simulink model "Pitch_shift_HDL"  (R2018b)
settings: Solver=FixedStepDiscrete  StartTime=0.0  StopTime=5  RelTol=1e-3
InitFcn:
  | load speech_signal
  | Fs = 48000;
  | Ts = 1/Fs;
  | 
  | FFT_size = 128;
  | FFT_size_half = FFT_size/2;
  | FFT_frame_shift = FFT_size/4;  % should be a power of two (to easily replace mode operator that is not HDL compatible)
  | FFT_frame_shift_Nbits = log2(FFT_frame_shift);
  | 
  | DPRAM1_size = FFT_size*2;  % number of words
  | DPRAM1_address_size = log2(DPRAM1_size);
  | 
  | 
  | 
  | SysRate_Upsample_Factor = 32;
  | 
  | 
  | Wbits = 32;    %fixdt(1,Wbits,Fbits)
  | Fbits = 28;
libraries: hdlsllib x16, simulink x5, dspxfrm3 x2, dspsigops x2
settings Model: Creator=Ross_admin  LastModifiedBy=Ross
settings OptimizationCC: BlockReduction=off  ConditionallyExecuteInputs=off  DefaultParameterBehavior=Inlined
settings DebuggingCC: AlgebraicLoopMsg=error  SingleTaskRateTransMsg=error
settings HardwareCC: ProdBitPerPointer=32  ProdBitPerSizeT=32  ProdBitPerPtrDiffT=32  ProdLargestAtomicFloat=None  ProdIntDivRoundTo=Undefined  ProdEndianess=Unspecified  ProdWordSize=32  ProdHWDeviceType=ASIC/FPGA->ASIC/FPGA  TargetBitPerPointer=64  TargetBitPerSizeT=64  TargetBitPerPtrDiffT=64  TargetLongLongMode=on  TargetIntDivRoundTo=Zero  TargetEndianess=LittleEndian  TargetWordSize=64  TargetHWDeviceType=Custom Processor->MATLAB Host Computer  ProdEqTarget=off
settings SFSimCC: SimUseLocalCustomCode=off
settings RTWCC: RTWUseLocalCustomCode=off
settings CodeAppCC: StateflowObjectComments=on

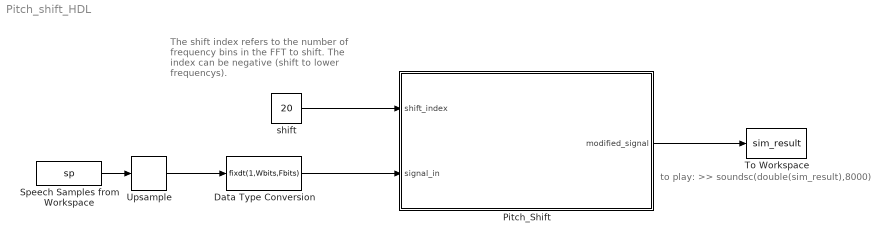
== system Pitch_shift_HDL ==
  note: The shift index refers to the number of
      | frequency bins in the FFT to shift.
      | The index can be negative
      | (shift to lower frequencys).
  note: to play: >> soundsc(double(sim_result),8000)
  Data Type Conversion : DataTypeConversion  OutDataTypeStr=fixdt(1,Wbits,Fbits)
  Pitch_Shift : Subsystem  TreatAsAtomicUnit=on
  Speech Samples from Workspace : FromWorkspace  VariableName=sp  SampleTime=Ts*6
  To Workspace : ToWorkspace  VariableName=sim_result  SampleTime=-1
  Upsample : dspsigops/Upsample  N=6  phase=0  RateOptions=Allow multirate processing  ic=0  mode=Unused parameter value
  shift : Constant  Value=20  OutDataTypeStr=fixdt(1,16,0)  SampleTime=Ts
  wires:
  Speech Samples from Workspace/1 -> Upsample/1
  Pitch_Shift/1(modified_signal) -> To Workspace/1
  Data Type Conversion/1 -> Pitch_Shift/2(signal_in)
  Upsample/1 -> Data Type Conversion/1
  shift/1 -> Pitch_Shift/1(shift_index)

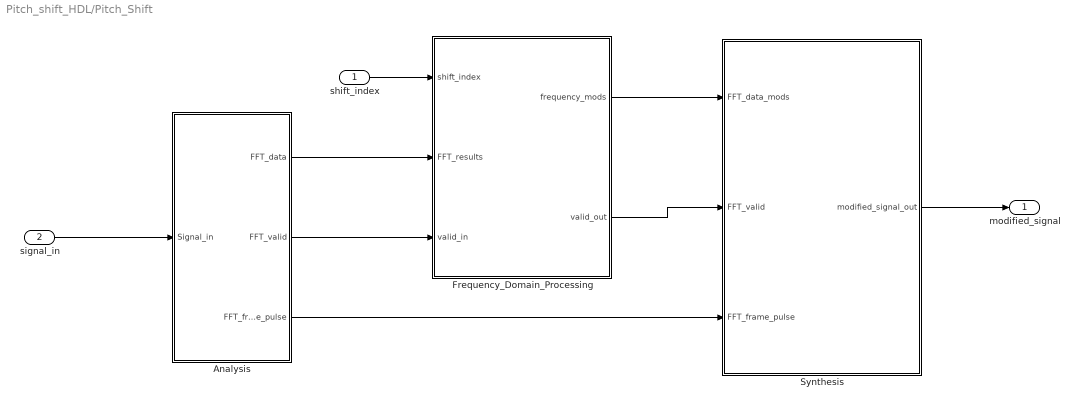
== system Pitch_shift_HDL/Pitch_Shift ==
  shift_index : Inport
  signal_in : Inport  Port=2
  Analysis : Subsystem
  Frequency_Domain_Processing : Subsystem
  Synthesis : Subsystem
  modified_signal : Outport
  wires:
  shift_index/1 -> Frequency_Domain_Processing/1(shift_index)
  signal_in/1 -> Analysis/1(Signal_in)
  Analysis/1(FFT_data) -> Frequency_Domain_Processing/2(FFT_results)
  Analysis/2(FFT_valid) -> Frequency_Domain_Processing/3(valid_in)
  Frequency_Domain_Processing/1(frequency_mods) -> Synthesis/1(FFT_data_mods)
  Frequency_Domain_Processing/2(valid_out) -> Synthesis/2(FFT_valid)
  Analysis/3(FFT_frame_pulse) -> Synthesis/3(FFT_frame_pulse)
  Synthesis/1(modified_signal_out) -> modified_signal/1

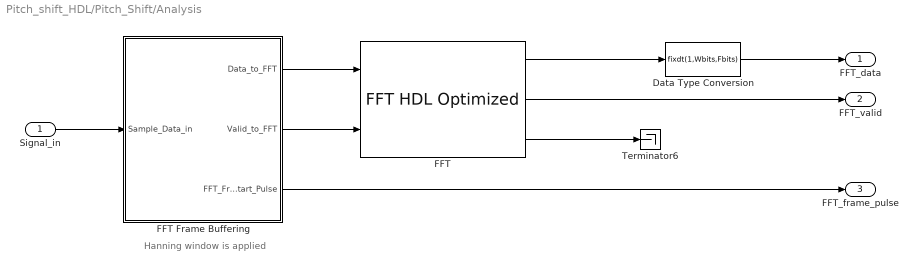
== system Pitch_shift_HDL/Pitch_Shift/Analysis ==
  note: Hanning window is applied
  Signal_in : Inport
  Data Type Conversion : DataTypeConversion  OutDataTypeStr=fixdt(1,Wbits,Fbits)
  FFT : dspxfrm3/FFT HDL Optimized  FFTLength=FFT_size  Architecture=Burst Radix 2  ComplexMultiplication=Use 4 multipliers and 2 adders  BitReversedOutput=off  BitReversedInput=off  Normalize=off  SimulateUsing=Code generation  RoundingMethod=Floor  ResetInputPort=off  StartOutputPort=off  EndOutputPort=off
      settings: SourceProductName=DSP System Toolbox  SourceProductBaseCode=DS
  FFT Frame Buffering : Subsystem
  Terminator6 : Terminator
  FFT_data : Outport
  FFT_valid : Outport  Port=2
  FFT_frame_pulse : Outport  Port=3
  wires:
  FFT/3 -> Terminator6/1
  FFT Frame Buffering/3(FFT_Frame_Start_Pulse) -> FFT_frame_pulse/1
  Signal_in/1 -> FFT Frame Buffering/1(Sample_Data_in)
  FFT Frame Buffering/2(Valid_to_FFT) -> FFT/2
  FFT Frame Buffering/1(Data_to_FFT) -> FFT/1
  Data Type Conversion/1 -> FFT_data/1
  FFT/2 -> FFT_valid/1
  FFT/1 -> Data Type Conversion/1

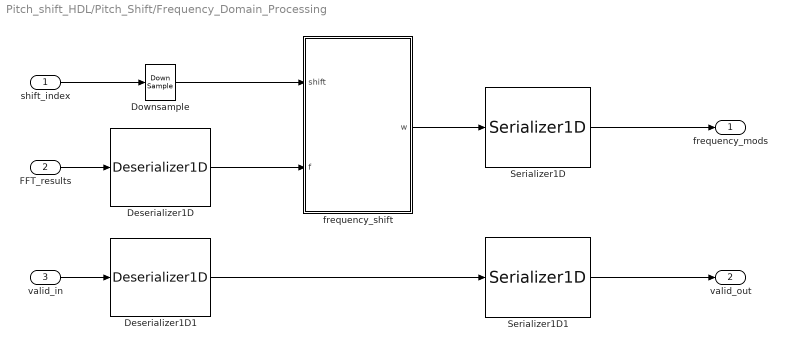
== system Pitch_shift_HDL/Pitch_Shift/Frequency_Domain_Processing ==
  shift_index : Inport
  FFT_results : Inport  Port=2
  valid_in : Inport  Port=3
  Deserializer1D : hdlsllib/HDL Operations/Deserializer1D  Ratio=FFT_size  IdleCycles=0  InitialCondition=0  startIn=off  validIn=off  validOut=off  inputDataDimensions=-1  inputSampleTime=-1  inputSignalType=auto
      settings: SourceProductName=HDL Coder  SourceProductBaseCode=HD
  Deserializer1D1 : hdlsllib/HDL Operations/Deserializer1D  Ratio=FFT_size  IdleCycles=0  InitialCondition=0  startIn=off  validIn=off  validOut=off  inputDataDimensions=-1  inputSampleTime=-1  inputSignalType=auto
      settings: SourceProductName=HDL Coder  SourceProductBaseCode=HD
  Downsample : DownSample  N=FFT_size/SysRate_Upsample_Factor  RateOptions=Allow multirate processing
  Serializer1D : hdlsllib/HDL Operations/Serializer1D  Ratio=FFT_size  IdleCycles=0  validIn=off  startOut=off  validOut=off  inputDataDimensions=-1  inputSampleTime=-1  inputSignalType=auto
      settings: SourceProductName=HDL Coder  SourceProductBaseCode=HD
  Serializer1D1 : hdlsllib/HDL Operations/Serializer1D  Ratio=FFT_size  IdleCycles=0  validIn=off  startOut=off  validOut=off  inputDataDimensions=-1  inputSampleTime=-1  inputSignalType=auto
      settings: SourceProductName=HDL Coder  SourceProductBaseCode=HD
  frequency_shift : MATLAB Function  TreatAsAtomicUnit=on
  frequency_mods : Outport
  valid_out : Outport  Port=2
  wires:
  Deserializer1D1/1 -> Serializer1D1/1
  Deserializer1D/1 -> frequency_shift/2(f)
  FFT_results/1 -> Deserializer1D/1
  frequency_shift/1(w) -> Serializer1D/1
  Serializer1D/1 -> frequency_mods/1
  valid_in/1 -> Deserializer1D1/1
  shift_index/1 -> Downsample/1
  Serializer1D1/1 -> valid_out/1
  Downsample/1 -> frequency_shift/1(shift)

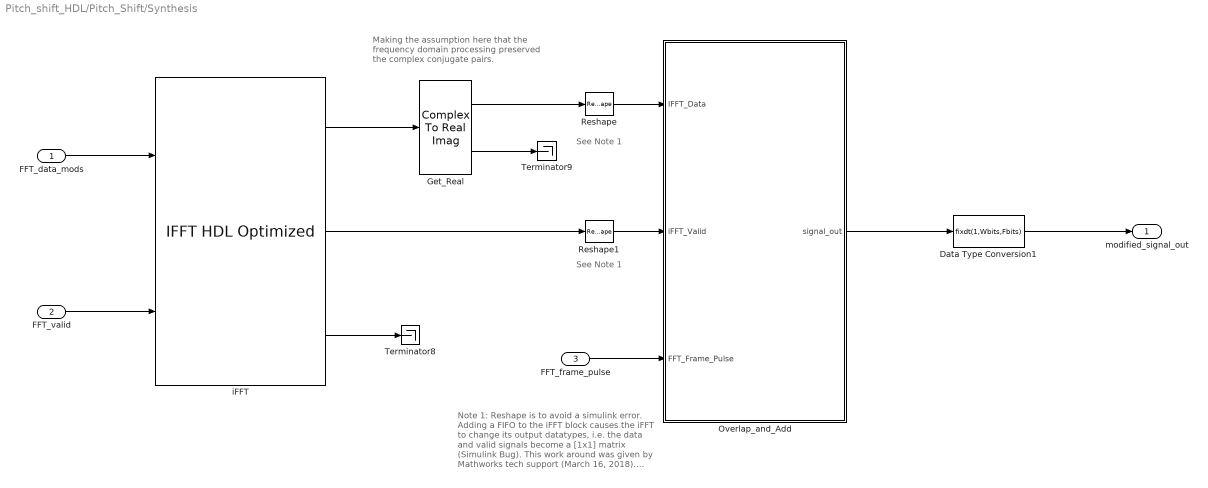
== system Pitch_shift_HDL/Pitch_Shift/Synthesis ==
  note: Making the assumption here
      | that the frequency domain processing
      | preserved the complex conjugate pairs.
  note: See Note 1
  note: Note 1:
      | Reshape is to avoid a simulink error.
      | Adding a FIFO to the iFFT block causes the
      | iFFT to change its output datatypes,
      | i.e. the data and valid signals
      | become a [1x1] matrix (Simulink Bug).
      | This work around was given by Mathworks
      | tech support (March 16, 2018).
      | Matlab 2017b
  note: See Note 1
  FFT_data_mods : Inport
  FFT_valid : Inport  Port=2
  FFT_frame_pulse : Inport  Port=3
  Data Type Conversion1 : DataTypeConversion  OutDataTypeStr=fixdt(1,Wbits,Fbits)
  Get_Real : ComplexToRealImag
  Overlap_and_Add : Subsystem
  Reshape : Reshape
  Reshape1 : Reshape
  Terminator8 : Terminator
  Terminator9 : Terminator
  iFFT : dspxfrm3/IFFT HDL Optimized  FFTLength=FFT_size  Architecture=Burst Radix 2  ComplexMultiplication=Use 4 multipliers and 2 adders  BitReversedOutput=off  BitReversedInput=off  Normalize=on  SimulateUsing=Code generation  RoundingMethod=Floor  ResetInputPort=off  StartOutputPort=off  EndOutputPort=off
      settings: SourceProductName=DSP System Toolbox  SourceProductBaseCode=DS
  modified_signal_out : Outport
  wires:
  iFFT/3 -> Terminator8/1
  Reshape1/1 -> Overlap_and_Add/2(iFFT_Valid)
  Reshape/1 -> Overlap_and_Add/1(IFFT_Data)
  iFFT/2 -> Reshape1/1
  Overlap_and_Add/1(signal_out) -> Data Type Conversion1/1
  FFT_data_mods/1 -> iFFT/1
  Data Type Conversion1/1 -> modified_signal_out/1
  iFFT/1 -> Get_Real/1
  Get_Real/1 -> Reshape/1
  Get_Real/2 -> Terminator9/1
  FFT_valid/1 -> iFFT/2
  FFT_frame_pulse/1 -> Overlap_and_Add/3(FFT_Frame_Pulse)

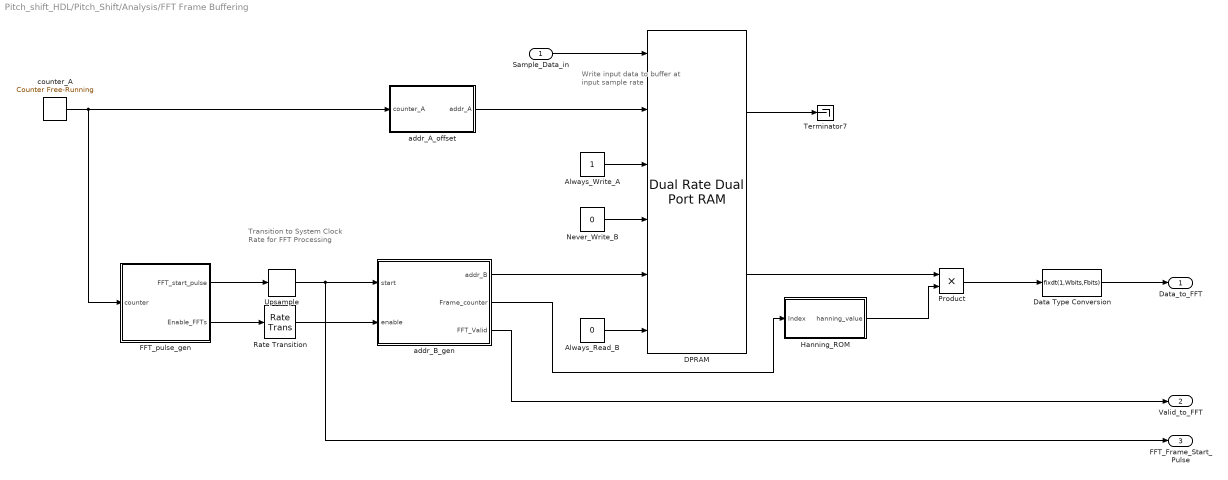
== system Pitch_shift_HDL/Pitch_Shift/Analysis/FFT Frame Buffering ==
  note: Transition to
      | System Clock Rate
      | for FFT Processing
  note: Write input data
      | to buffer at input
      | sample rate
  Sample_Data_in : Inport
  Always_Read_B : Constant  Value=0  OutDataTypeStr=boolean  SampleTime=Ts/SysRate_Upsample_Factor
  Always_Write_A : Constant  OutDataTypeStr=boolean  SampleTime=Ts
  DPRAM : hdlsllib/HDL RAMs/Dual Rate Dual Port RAM  ram_size=DPRAM1_address_size
      settings: SourceProductName=HDL Coder  SourceProductBaseCode=HD
  Data Type Conversion : DataTypeConversion  OutDataTypeStr=fixdt(1,Wbits,Fbits)
  FFT_pulse_gen : Subsystem
  Hanning_ROM : Subsystem
  Never_Write_B : Constant  Value=0  OutDataTypeStr=fixdt(1,Wbits,Fbits)  SampleTime=Ts/SysRate_Upsample_Factor
  Product : Product
  Rate Transition : RateTransition  OutPortSampleTimeOpt=Multiple of input port sample time  OutPortSampleTimeMultiple=1/SysRate_Upsample_Factor
  Terminator7 : Terminator
  Upsample : dspsigops/Upsample  N=SysRate_Upsample_Factor  phase=0  RateOptions=Allow multirate processing  ic=0  mode=Unused parameter value
  addr_A_offset : Subsystem
  addr_B_gen : Subsystem
  counter_A : simulink/Sources/Counter Free-Running  NumBits=DPRAM1_address_size  tsamp=Ts
  Data_to_FFT : Outport
  Valid_to_FFT : Outport  Port=2
  FFT_Frame_Start_Pulse : Outport  Port=3
  wires:
  Always_Write_A/1 -> DPRAM/3
  Never_Write_B/1 -> DPRAM/4
  Always_Read_B/1 -> DPRAM/6
  DPRAM/1 -> Terminator7/1
  addr_B_gen/3(FFT_Valid) -> Valid_to_FFT/1
  addr_B_gen/1(addr_B) -> DPRAM/5
  counter_A/1 -> addr_A_offset/1(counter_A), FFT_pulse_gen/1(counter)
  Sample_Data_in/1 -> DPRAM/1
  addr_A_offset/1(addr_A) -> DPRAM/2
  addr_B_gen/2(Frame_counter) -> Hanning_ROM/1(Index)
  Product/1 -> Data Type Conversion/1
  DPRAM/2 -> Product/1
  Hanning_ROM/1(hanning_value) -> Product/2
  Data Type Conversion/1 -> Data_to_FFT/1
  Rate Transition/1 -> addr_B_gen/2(enable)
  FFT_pulse_gen/1(FFT_start_pulse) -> Upsample/1
  FFT_pulse_gen/2(Enable_FFTs) -> Rate Transition/1
  Upsample/1 -> FFT_Frame_Start_Pulse/1, addr_B_gen/1(start)

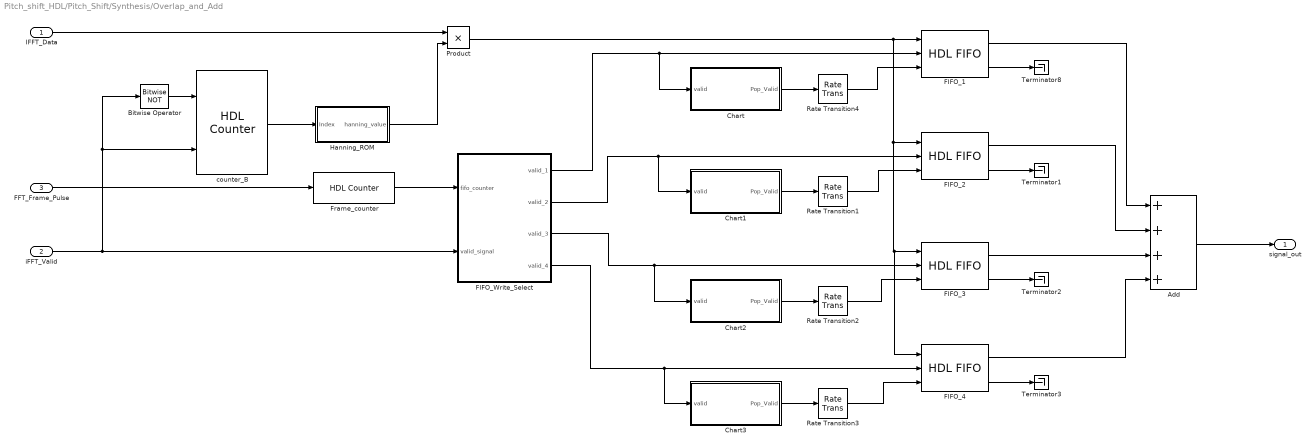
== system Pitch_shift_HDL/Pitch_Shift/Synthesis/Overlap_and_Add ==
  IFFT_Data : Inport
  iFFT_Valid : Inport  Port=2
  FFT_Frame_Pulse : Inport  Port=3
  Add : Sum  Inputs=4
  Bitwise Operator : simulink/Logic and Bit Operations/Bitwise Operator  logicop=NOT  UseBitMask=off  BitMask=bin2dec('11011001')  BitMaskRealWorld=Stored Integer
  Chart : Stateflow chart  TreatAsAtomicUnit=on
  Chart1 : Stateflow chart  TreatAsAtomicUnit=on
  Chart2 : Stateflow chart  TreatAsAtomicUnit=on
  Chart3 : Stateflow chart  TreatAsAtomicUnit=on
  FIFO_{1..4} (4 alike) : hdlsllib/HDL RAMs/HDL FIFO  fifo_size=FFT_size  ratio=SysRate_Upsample_Factor  push_msg=Warning  pop_msg=Warning  show_empty=off  show_full=on  show_num=off
      settings: SourceProductName=HDL Coder  SourceProductBaseCode=HD
  FIFO_Write_Select : MATLAB Function  TreatAsAtomicUnit=on
  Frame_counter : hdlsllib/Sources/HDL Counter  CountType=Free running  CountInit=2  CountStep=1  CountMax=1024  CountFromType=Initial value  CountFrom=2  CountResetPort=off  CountLoadPort=off  CountEnbPort=on  CountDirPort=off  CountDataType=Unsigned  CountWordLen=2  CountFracLen=0  CountSampTime=1
      settings: SourceProductBaseCode=HD
  Hanning_ROM : Subsystem
  Product : Product
  Rate Transition{1..4} (4 alike) : RateTransition  OutPortSampleTimeOpt=Multiple of input port sample time  OutPortSampleTimeMultiple=SysRate_Upsample_Factor
  Terminator{1..3,8} (4 alike) : Terminator
  counter_B : hdlsllib/Sources/HDL Counter  CountType=Count limited  CountInit=0  CountStep=1  CountMax=FFT_size  CountFromType=Initial value  CountFrom=0  CountResetPort=on  CountLoadPort=off  CountEnbPort=on  CountDirPort=off  CountDataType=Unsigned  CountWordLen=DPRAM1_address_size  CountFracLen=0  CountSampTime=1
      settings: SourceProductBaseCode=HD
  signal_out : Outport
  wires:
  FIFO_1/1 -> Add/1
  FIFO_3/1 -> Add/3
  FFT_Frame_Pulse/1 -> Frame_counter/1
  FIFO_2/1 -> Add/2
  FIFO_Write_Select/3(valid_3) -> Chart2/1(valid), FIFO_3/2
  FIFO_Write_Select/4(valid_4) -> Chart3/1(valid), FIFO_4/2
  FIFO_4/1 -> Add/4
  FIFO_Write_Select/1(valid_1) -> FIFO_1/2, Chart/1(valid)
  FIFO_Write_Select/2(valid_2) -> FIFO_2/2, Chart1/1(valid)
  Add/1 -> signal_out/1
  Frame_counter/1 -> FIFO_Write_Select/1(fifo_counter)
  FIFO_4/2 -> Terminator3/1
  FIFO_2/2 -> Terminator1/1
  FIFO_3/2 -> Terminator2/1
  Bitwise Operator/1 -> counter_B/1
  iFFT_Valid/1 -> counter_B/2, Bitwise Operator/1, FIFO_Write_Select/2(valid_signal)
  IFFT_Data/1 -> Product/1
  Product/1 -> FIFO_4/1, FIFO_3/1, FIFO_2/1, FIFO_1/1
  Hanning_ROM/1(hanning_value) -> Product/2
  counter_B/1 -> Hanning_ROM/1(Index)
  Chart/1(Pop_Valid) -> Rate Transition4/1
  Rate Transition4/1 -> FIFO_1/3
  FIFO_1/2 -> Terminator8/1
  Chart1/1(Pop_Valid) -> Rate Transition1/1
  Rate Transition1/1 -> FIFO_2/3
  Chart2/1(Pop_Valid) -> Rate Transition2/1
  Rate Transition2/1 -> FIFO_3/3
  Chart3/1(Pop_Valid) -> Rate Transition3/1
  Rate Transition3/1 -> FIFO_4/3

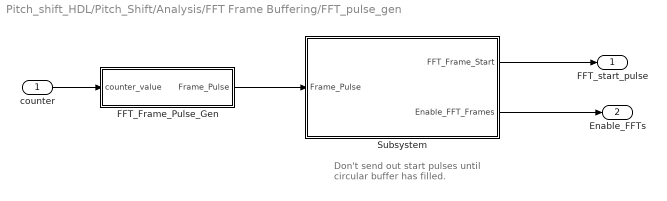
== system Pitch_shift_HDL/Pitch_Shift/Analysis/FFT Frame Buffering/FFT_pulse_gen ==
  note: Don't send out start pulses until
      | circular buffer has filled.
  counter : Inport
  FFT_Frame_Pulse_Gen : Subsystem
  Subsystem : Subsystem
  FFT_start_pulse : Outport
  Enable_FFTs : Outport  Port=2
  wires:
  counter/1 -> FFT_Frame_Pulse_Gen/1("counter_value ")
  Subsystem/1(FFT_Frame_Start) -> FFT_start_pulse/1
  Subsystem/2(Enable_FFT_Frames) -> Enable_FFTs/1
  FFT_Frame_Pulse_Gen/1(Frame_Pulse) -> Subsystem/1(Frame_Pulse)

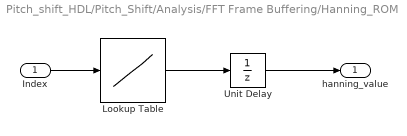
== system Pitch_shift_HDL/Pitch_Shift/Analysis/FFT Frame Buffering/Hanning_ROM ==
  Index : Inport
  Lookup Table : Lookup_n-D  NumberOfTableDimensions=1  BreakpointsForDimension1=[0:FFT_size]  IndexSearchMethod=Evenly spaced points  Table=hanning(FFT_size+1)  InterpMethod=Flat  ExtrapMethod=Clip  DiagnosticForOutOfRangeInput=Error  UseLastTableValue=on  OutDataTypeStr=fixdt(1,24,22)  RndMeth=Simplest  InputSameDT=on
  Unit Delay : UnitDelay  SampleTime=-1
  hanning_value : Outport
  wires:
  Unit Delay/1 -> hanning_value/1
  Index/1 -> Lookup Table/1
  Lookup Table/1 -> Unit Delay/1

== system Pitch_shift_HDL/Pitch_Shift/Analysis/FFT Frame Buffering/addr_A_offset ==
  note: Add 1 to counter since the read pointer (addr_B)
      | can catch the write pointer (addr_A) if
      | SysRate_Upsample_Factor is large enough
  counter_A : Inport
  Add : Sum  OutDataTypeStr=fixdt(0,DPRAM1_address_size,0)
  write_offset : Constant  OutDataTypeStr=fixdt(0,DPRAM1_address_size,0)  SampleTime=Ts
  addr_A : Outport
  wires:
  write_offset/1 -> Add/2
  Add/1 -> addr_A/1
  counter_A/1 -> Add/1

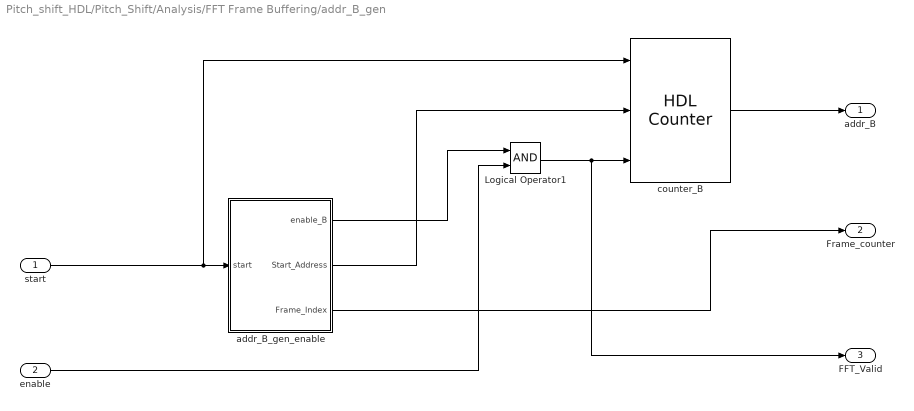
== system Pitch_shift_HDL/Pitch_Shift/Analysis/FFT Frame Buffering/addr_B_gen ==
  start : Inport
  enable : Inport  Port=2
  Logical Operator1 : Logic  AllPortsSameDT=off  OutDataTypeStr=boolean
  addr_B_gen_enable : Subsystem
  counter_B : hdlsllib/Sources/HDL Counter  CountType=Free running  CountInit=DPRAM1_size-10  CountStep=1  CountMax=1024  CountFromType=Initial value  CountFrom=DPRAM1_size-10  CountResetPort=off  CountLoadPort=on  CountEnbPort=on  CountDirPort=off  CountDataType=Unsigned  CountWordLen=DPRAM1_address_size  CountFracLen=0  CountSampTime=1
      settings: SourceProductBaseCode=HD
  addr_B : Outport
  Frame_counter : Outport  Port=2
  FFT_Valid : Outport  Port=3
  wires:
  counter_B/1 -> addr_B/1
  start/1 -> counter_B/1, addr_B_gen_enable/1(start)
  addr_B_gen_enable/1(enable_B) -> Logical Operator1/1
  addr_B_gen_enable/2(Start_Address) -> counter_B/2
  enable/1 -> Logical Operator1/2
  addr_B_gen_enable/3(Frame_Index) -> Frame_counter/1
  Logical Operator1/1 -> FFT_Valid/1, counter_B/3

== system Pitch_shift_HDL/Pitch_Shift/Synthesis/Overlap_and_Add/Hanning_ROM ==
  Index : Inport
  Lookup Table : Lookup_n-D  NumberOfTableDimensions=1  BreakpointsForDimension1=[0:FFT_size]  IndexSearchMethod=Evenly spaced points  Table=hanning(FFT_size+1)  InterpMethod=Flat  ExtrapMethod=Clip  DiagnosticForOutOfRangeInput=Error  UseLastTableValue=on  OutDataTypeStr=fixdt(1,24,22)  RndMeth=Simplest  InputSameDT=on
  Unit Delay : UnitDelay  SampleTime=-1
  hanning_value : Outport
  wires:
  Unit Delay/1 -> hanning_value/1
  Index/1 -> Lookup Table/1
  Lookup Table/1 -> Unit Delay/1

== system Pitch_shift_HDL/Pitch_Shift/Analysis/FFT Frame Buffering/FFT_pulse_gen/FFT_Frame_Pulse_Gen ==
  "counter_value " : Inport
  Bit Slice : hdlsllib/Logic and Bit Operations/Bit Slice  lidx=log2(FFT_frame_shift)-1  ridx=0
  Compare To Zero : simulink/Logic and Bit Operations/Compare To Zero  relop===  OutDataTypeStr=boolean
  Frame_Pulse : Outport
  wires:
  "counter_value "/1 -> Bit Slice/1
  Compare To Zero/1 -> Frame_Pulse/1
  Bit Slice/1 -> Compare To Zero/1

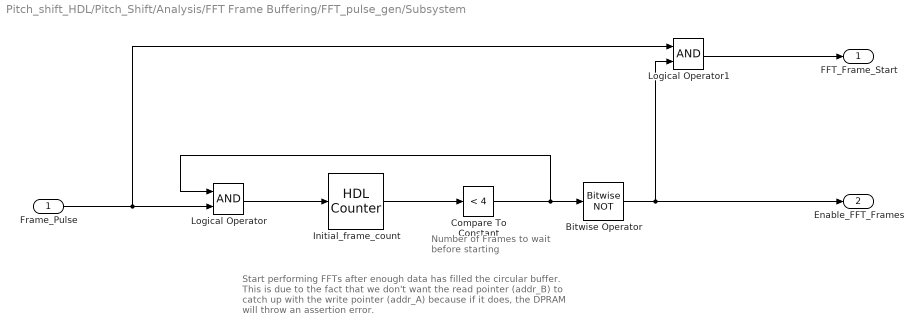
== system Pitch_shift_HDL/Pitch_Shift/Analysis/FFT Frame Buffering/FFT_pulse_gen/Subsystem ==
  note: Number of Frames
      | to wait before starting
  note: Start performing FFTs after enough data has filled the circular buffer.
      | This is due to the fact that we don't want the read pointer (addr_B)
      | to catch up with the  write pointer (addr_A) because if it does,
      | the DPRAM will throw an assertion error.
  Frame_Pulse : Inport
  Bitwise Operator : simulink/Logic and Bit Operations/Bitwise Operator  logicop=NOT  UseBitMask=off  BitMask=bin2dec('11011001')  BitMaskRealWorld=Stored Integer
  Compare To Constant : simulink/Logic and Bit Operations/Compare To Constant  relop=<  const=4  OutDataTypeStr=boolean
  Initial_frame_count : hdlsllib/Sources/HDL Counter  CountType=Count limited  CountInit=0  CountStep=1  CountMax=4  CountFromType=Specify  CountFrom=0  CountResetPort=off  CountLoadPort=off  CountEnbPort=on  CountDirPort=off  CountDataType=Unsigned  CountWordLen=5  CountFracLen=0  CountSampTime=1
      settings: SourceProductBaseCode=HD
  Logical Operator : Logic  AllPortsSameDT=off  OutDataTypeStr=boolean
  Logical Operator1 : Logic  AllPortsSameDT=off  OutDataTypeStr=boolean
  FFT_Frame_Start : Outport
  Enable_FFT_Frames : Outport  Port=2
  wires:
  Logical Operator1/1 -> FFT_Frame_Start/1
  Frame_Pulse/1 -> Logical Operator/2, Logical Operator1/1
  Initial_frame_count/1 -> Compare To Constant/1
  Logical Operator/1 -> Initial_frame_count/1
  Compare To Constant/1 -> Bitwise Operator/1, Logical Operator/1
  Bitwise Operator/1 -> Enable_FFT_Frames/1, Logical Operator1/2

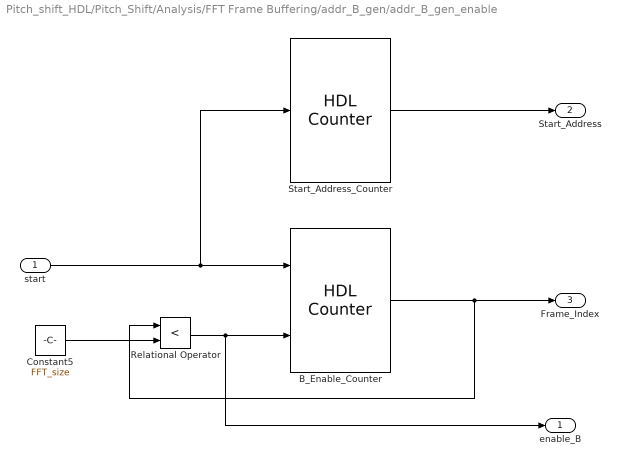
== system Pitch_shift_HDL/Pitch_Shift/Analysis/FFT Frame Buffering/addr_B_gen/addr_B_gen_enable ==
  start : Inport
  B_Enable_Counter : hdlsllib/Sources/HDL Counter  CountType=Count limited  CountInit=0  CountStep=1  CountMax=FFT_size  CountFromType=Specify  CountFrom=0  CountResetPort=on  CountLoadPort=off  CountEnbPort=on  CountDirPort=off  CountDataType=Unsigned  CountWordLen=DPRAM1_address_size  CountFracLen=0  CountSampTime=1
      settings: SourceProductBaseCode=HD
  Constant5 : Constant  Value=FFT_size  OutDataTypeStr=fixdt(0,11,0)  SampleTime=Ts/SysRate_Upsample_Factor
  Relational Operator : RelationalOperator  Operator=<  OutDataTypeStr=boolean  ZeroCross=off  RndMeth=Nearest
  Start_Address_Counter : hdlsllib/Sources/HDL Counter  CountType=Free running  CountInit=0  CountStep=FFT_frame_shift  CountMax=DPRAM1_size  CountFromType=Initial value  CountFrom=0  CountResetPort=off  CountLoadPort=off  CountEnbPort=on  CountDirPort=off  CountDataType=Unsigned  CountWordLen=DPRAM1_address_size  CountFracLen=0  CountSampTime=1
      settings: SourceProductBaseCode=HD
  enable_B : Outport
  Start_Address : Outport  Port=2
  Frame_Index : Outport  Port=3
  wires:
  Relational Operator/1 -> enable_B/1, B_Enable_Counter/2
  Constant5/1 -> Relational Operator/2
  B_Enable_Counter/1 -> Frame_Index/1, Relational Operator/1
  start/1 -> Start_Address_Counter/1, B_Enable_Counter/1
  Start_Address_Counter/1 -> Start_Address/1

== stateflow chart Pitch_shift_HDL/Pitch_Shift/Synthesis/Overlap_and_Add/Chart1 ==
  settings: executeAtInitialization=1
  state valid_high
    entry: Pop_Valid=fi(0,0,1,0);
  state Pop_assert
    entry: Pop_Valid=fi(1,0,1,0);
  state valid_low
    entry: Pop_Valid=fi(0,0,1,0);
  state Start_up
    entry: Pop_Valid=fi(0,0,1,0);
  (default) -> Start_up
  Start_up -> valid_low : [valid == 0]
  valid_high -> Pop_assert [order 1] : [valid == 0]
  valid_low -> valid_high [order 1] : [valid == 1]
  valid_low -> valid_low [order 2] : [valid == 0]
  valid_high -> valid_high [order 2] : [valid == 1]
  data: valid input; Pop_Valid output

== matlab function Pitch_shift_HDL/Pitch_Shift/Synthesis/Overlap_and_Add/FIFO_Write_Select ==
  data: fifo_counter input; valid_1 output; valid_signal input; valid_2 output; valid_3 output; valid_4 output
function [valid_1, valid_2, valid_3, valid_4] = fcn(fifo_counter, valid_signal)
%#codegen



switch fifo_counter
    case 0
        valid_1 = valid_signal;
        valid_2 = false;
        valid_3 = false;
        valid_4 = false;
    case 1
        valid_1 = false;
        valid_2 = valid_signal;
        valid_3 = false;
        valid_4 = false;
    case 2
        valid_1 = false;
        valid_2 = false;
        valid_3 = valid_signal;
        valid_4 = false;
    case 3
        valid_1 = false;
        valid_2 = false;
        valid_3 = false;
        valid_4 = valid_signal;
    otherwise
        valid_1 = false;
        valid_2 = false;
        valid_3 = false;
        valid_4 = false;
       
end

== stateflow chart Pitch_shift_HDL/Pitch_Shift/Synthesis/Overlap_and_Add/Chart2 ==
  settings: executeAtInitialization=1
  state valid_high
    entry: Pop_Valid=fi(0,0,1,0);
  state Pop_assert
    entry: Pop_Valid=fi(1,0,1,0);
  state valid_low
    entry: Pop_Valid=fi(0,0,1,0);
  state Start_up
    entry: Pop_Valid=fi(0,0,1,0);
  (default) -> Start_up
  Start_up -> valid_low : [valid == 0]
  valid_high -> Pop_assert [order 1] : [valid == 0]
  valid_low -> valid_high [order 1] : [valid == 1]
  valid_low -> valid_low [order 2] : [valid == 0]
  valid_high -> valid_high [order 2] : [valid == 1]
  data: valid input; Pop_Valid output

== stateflow chart Pitch_shift_HDL/Pitch_Shift/Synthesis/Overlap_and_Add/Chart3 ==
  settings: executeAtInitialization=1
  state valid_high
    entry: Pop_Valid=fi(0,0,1,0);
  state Pop_assert
    entry: Pop_Valid=fi(1,0,1,0);
  state valid_low
    entry: Pop_Valid=fi(0,0,1,0);
  state Start_up
    entry: Pop_Valid=fi(0,0,1,0);
  (default) -> Start_up
  Start_up -> valid_low : [valid == 0]
  valid_high -> Pop_assert [order 1] : [valid == 0]
  valid_low -> valid_high [order 1] : [valid == 1]
  valid_low -> valid_low [order 2] : [valid == 0]
  valid_high -> valid_high [order 2] : [valid == 1]
  data: valid input; Pop_Valid output

== matlab function Pitch_shift_HDL/Pitch_Shift/Frequency_Domain_Processing/frequency_shift ==
  data: shift input; f input; w output
function w = fcn(shift,f)

Wbits = 32;
Fbits = 28;



N = length(f);
Nd2 = N/2;
w = fi(complex(zeros(N,1)), 1, Wbits, Fbits);

if shift == 0
    w = f;
else
        
    w(1)     = fi(complex(0), 1, Wbits, Fbits);   % we don't care about dc term (in fact it is better if we eliminate it)
    w(Nd2+1) = fi(complex(0), 1, Wbits, Fbits);   % just zero frequency at +-pi since both positive and negative frequencies map here when shifted (simplification)
        
    if shift > 0  % increase the frequencies
        
        for i=2:Nd2  % shift positive frequencies to the right
            if i <= shift
                w(i) = fi(complex(0), 1, Wbits, Fbits); % fill in vacated positive frequencies with zeros
            else
                w(i) = f(i-shift);
            end    
        end
        for i=N:-1:Nd2+2  % shift negative frequencies to the left
            if i > N-shift
                w(i) = fi(complex(0), 1, Wbits, Fbits); % fill in vacated negative frequencies with zeros
            else
                w(i) = f(i+shift);
            end    
        end
        
    end
                
    if shift < 0  % decrease the frequencies
      
        for i=Nd2:-1:2  % shift positive frequencies to the left
            if i > Nd2-shift
                w(i) = fi(complex(0), 1, Wbits, Fbits); % fill in vacated positive frequencies with zeros
            else
                %[i i+shift]
                w(i) = f(i-shift);
            end    
        end
        
        for i=Nd2+2:N  % shift negative frequencies to the right
            if i <= Nd2+2+shift
                w(i) = fi(complex(0), 1, Wbits, Fbits); % fill in vacated negative frequencies with zeros
            else
                w(i) = f(i+shift);
            end    
        end
        


    end
end

== stateflow chart Pitch_shift_HDL/Pitch_Shift/Synthesis/Overlap_and_Add/Chart ==
  settings: executeAtInitialization=1
  state valid_high
    entry: Pop_Valid=fi(0,0,1,0);
  state Pop_assert
    entry: Pop_Valid=fi(1,0,1,0);
  state valid_low
    entry: Pop_Valid=fi(0,0,1,0);
  state Start_up
    entry: Pop_Valid=fi(0,0,1,0);
  (default) -> Start_up
  Start_up -> valid_low : [valid == 0]
  valid_high -> Pop_assert [order 1] : [valid == 0]
  valid_low -> valid_high [order 1] : [valid == 1]
  valid_low -> valid_low [order 2] : [valid == 0]
  valid_high -> valid_high [order 2] : [valid == 1]
  data: valid input; Pop_Valid output
